simulink model "confronto_lineare_non_lineare_retroazione_gradino"  (R2018a)
settings: Solver=VariableStepAuto  StartTime=0.0  StopTime=100  RelTol=1e-3
undefined symbols (not defined in the file): A, alpha_eq, B, dati, fd, fd_eq, K, x0, x_eq
settings Model: Creator=Ivonne  LastModifiedBy=Ivonne

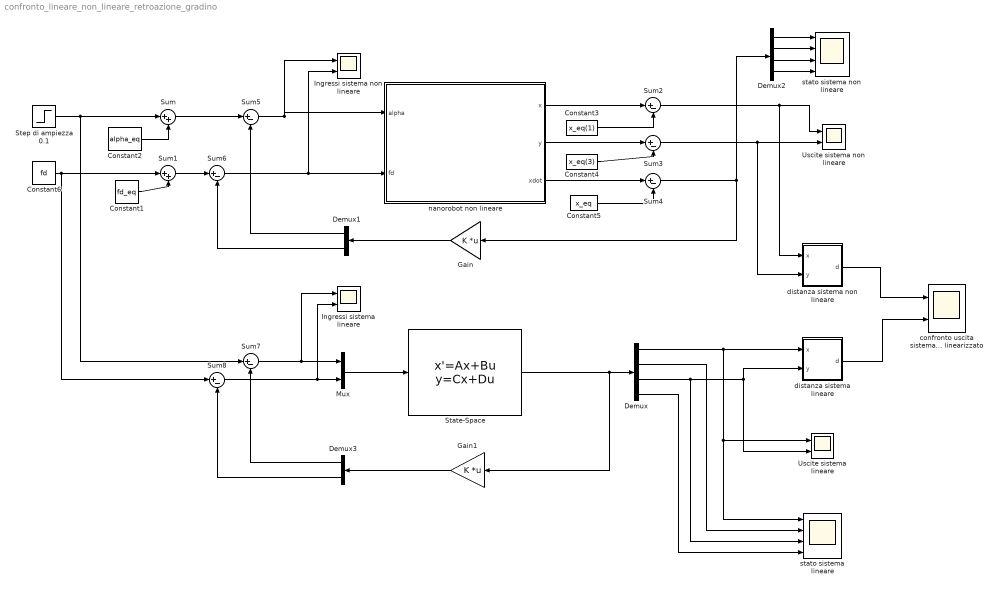
== system confronto_lineare_non_lineare_retroazione_gradino ==
  Constant1 : Constant  Value=fd_eq
  Constant2 : Constant  Value=alpha_eq
  Constant3 : Constant  Value=x_eq(1)
  Constant4 : Constant  Value=x_eq(3)
  Constant5 : Constant  Value=x_eq
  Constant6 : Constant  Value=fd
  Demux : Demux
  Demux1 : Demux  Outputs=2
  Demux2 : Demux
  Demux3 : Demux  Outputs=2
  Gain : Gain  Gain=K  Multiplication=Matrix(K*u)
  Gain1 : Gain  Gain=K  Multiplication=Matrix(K*u)
  Ingressi sistema lineare : Scope  NumInputPorts=2
  Ingressi sistema non lineare : Scope  NumInputPorts=2
  Mux : Mux  Inputs=2
  State-Space : StateSpace  A=A  B=B  C=eye(4)  D=zeros(4,2)  InitialCondition=x0
  Step di ampiezza 0.1 : Step  Time=0.1  After=0.1  SampleTime=0
  Sum : Sum  Inputs=|++
  Sum1 : Sum  Inputs=|++
  Sum{2..8} (7 alike) : Sum  Inputs=|+-
  Uscite sistema lineare : Scope  NumInputPorts=2
  Uscite sistema non lineare : Scope  NumInputPorts=2
  confronto uscita sistema non lineare e modello linearizzato : Scope  NumInputPorts=2
  "distanza sistema non lineare " : Subsystem
  distanza sistema lineare : Subsystem
  nanorobot non lineare : Subsystem
  stato sistema lineare : Scope  NumInputPorts=4
  stato sistema non lineare : Scope  NumInputPorts=4
  wires:
  Constant2/1 -> Sum/2
  Constant1/1 -> Sum1/2
  "distanza sistema non lineare "/1(d) -> confronto uscita sistema non lineare e modello linearizzato/1
  Mux/1 -> State-Space/1
  State-Space/1 -> Gain1/1, Demux/1
  distanza sistema lineare/1(d) -> confronto uscita sistema non lineare e modello linearizzato/2
  Constant3/1 -> Sum2/2
  nanorobot non lineare/1(x) -> Sum2/1
  Sum2/1 -> "distanza sistema non lineare "/1(x), Uscite sistema non lineare/1
  nanorobot non lineare/2(y) -> Sum3/1
  Constant4/1 -> Sum3/2
  Sum3/1 -> "distanza sistema non lineare "/2(y), Uscite sistema non lineare/2
  Step di ampiezza 0.1/1 -> Sum7/1, Sum/1
  nanorobot non lineare/3(xdot) -> Sum4/1
  Constant5/1 -> Sum4/2
  Demux2/4 -> stato sistema non lineare/4
  Demux2/1 -> stato sistema non lineare/1
  Demux2/2 -> stato sistema non lineare/2
  Demux2/3 -> stato sistema non lineare/3
  Sum/1 -> Sum5/1
  Sum1/1 -> Sum6/1
  Sum5/1 -> nanorobot non lineare/1(alpha), Ingressi sistema non lineare/1
  Sum6/1 -> nanorobot non lineare/2(fd), Ingressi sistema non lineare/2
  Gain/1 -> Demux1/1
  Demux1/1 -> Sum5/2
  Demux1/2 -> Sum6/2
  Sum7/1 -> Mux/1, Ingressi sistema lineare/1
  Sum8/1 -> Ingressi sistema lineare/2, Mux/2
  Gain1/1 -> Demux3/1
  Demux3/1 -> Sum7/2
  Demux3/2 -> Sum8/2
  Demux/1 -> stato sistema lineare/1, Uscite sistema lineare/1, distanza sistema lineare/1(x)
  Demux/3 -> stato sistema lineare/3, Uscite sistema lineare/2, distanza sistema lineare/2(y)
  Demux/2 -> stato sistema lineare/2
  Demux/4 -> stato sistema lineare/4
  Sum4/1 -> Gain/1, Demux2/1
  Constant6/1 -> Sum1/1, Sum8/1

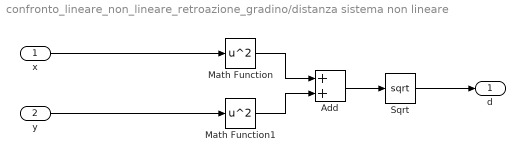
== system confronto_lineare_non_lineare_retroazione_gradino/distanza sistema non lineare  ==
  x : Inport
  y : Inport  Port=2
  Add : Sum
  Math Function : Math  Operator=square  SaturateOnIntegerOverflow=on
  Math Function1 : Math  Operator=square  SaturateOnIntegerOverflow=on
  Sqrt : Sqrt  SaturateOnIntegerOverflow=on
  d : Outport
  wires:
  Add/1 -> Sqrt/1
  x/1 -> Math Function/1
  Math Function/1 -> Add/1
  Math Function1/1 -> Add/2
  Sqrt/1 -> d/1
  y/1 -> Math Function1/1

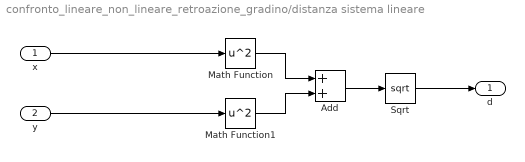
== system confronto_lineare_non_lineare_retroazione_gradino/distanza sistema lineare ==
  x : Inport
  y : Inport  Port=2
  Add : Sum
  Math Function : Math  Operator=square  SaturateOnIntegerOverflow=on
  Math Function1 : Math  Operator=square  SaturateOnIntegerOverflow=on
  Sqrt : Sqrt  SaturateOnIntegerOverflow=on
  d : Outport
  wires:
  Add/1 -> Sqrt/1
  x/1 -> Math Function/1
  Math Function/1 -> Add/1
  Math Function1/1 -> Add/2
  Sqrt/1 -> d/1
  y/1 -> Math Function1/1

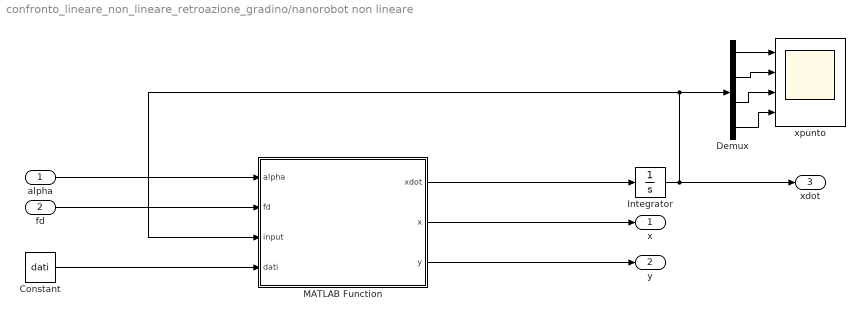
== system confronto_lineare_non_lineare_retroazione_gradino/nanorobot non lineare ==
  alpha : Inport
  fd : Inport  Port=2
  Constant : Constant  Value=dati
  Demux : Demux
  Integrator : Integrator  InitialCondition=x0
  MATLAB Function : MATLAB Function  TreatAsAtomicUnit=on
  xpunto : Scope  NumInputPorts=4
  x : Outport
  y : Outport  Port=2
  xdot : Outport  Port=3
  wires:
  MATLAB Function/1(xdot) -> Integrator/1
  Integrator/1 -> xdot/1, MATLAB Function/3(input), Demux/1
  MATLAB Function/2(x) -> x/1
  Constant/1 -> MATLAB Function/4(dati)
  alpha/1 -> MATLAB Function/1(alpha)
  Demux/1 -> xpunto/1
  Demux/2 -> xpunto/2
  Demux/3 -> xpunto/3
  Demux/4 -> xpunto/4
  MATLAB Function/3(y) -> y/1
  fd/1 -> MATLAB Function/2(fd)

== matlab function confronto_lineare_non_lineare_retroazione_gradino/nanorobot non lineare/MATLAB Function ==
  data: xdot output; alpha input; fd input; input input; x output; dati input; y output
function [ xdot, x, y ] = fcn(alpha, fd, input, dati)
% input : condizioni iniziali
% u : ingresso del sistema -> [ alpha, fd]
% dati : parametri del modello fisico -> [ R, Fm, m, eta,l, dP, r, vf ]
R= dati(1);                 
Fm = dati(2);  
m = dati(3);
eta = dati(4);
l = dati(5);
dP = dati(6);
r = dati(7);
vf = dati(8);
% variabili di stato 
% x1 = x, x2 = xp -> x1p, x3 = y, x4 = yp -> x3p
% allora xpp = x2p e ypp = x4p
x1 = input(1); % xdot(1) = x2 -> 1/s 
x2 = input(2); % xdot(2) = x2p -> 1/s 
x3 = input(3); % xdot(3) = x4 -> 1/s
x4 = input(4); % xdot(4) = x4p -> 1/s
% forma di stato
xdot = [ x2;
         ((-6*pi*eta*R)/m)*x2 + ((6*pi*eta*R)/m)*vf + (Fm/m)*cos(alpha) + fd/m;
         x4;
         ((-6*pi*eta*R)/m)*x4 + (Fm/m)*sin(alpha)];

% coordinate cartesiane
x = x1;
y = x3;
